simulink library "Rishi_Library"  (R2023a)
settings: Solver=VariableStepAuto  StartTime=0.0  StopTime=10.0  RelTol=1e-3

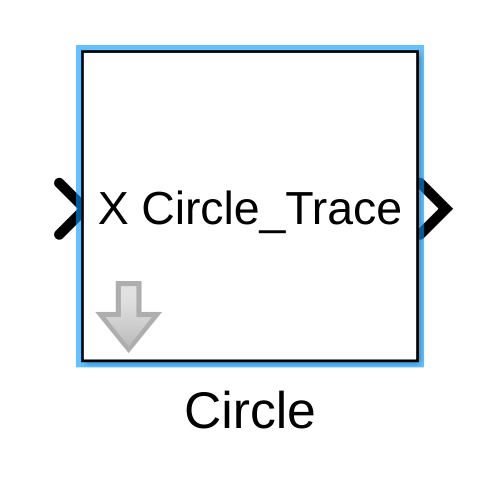
[thumbnail: Simulink's stored preview of the top-level diagram]
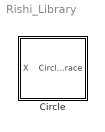
== system Rishi_Library ==
  Circle : Subsystem  mask{X_Offset=0, Y_Offset=0, Radius=0}
      mask prompts: X_Offset "X Offset"; Y_Offset "Y Offset"

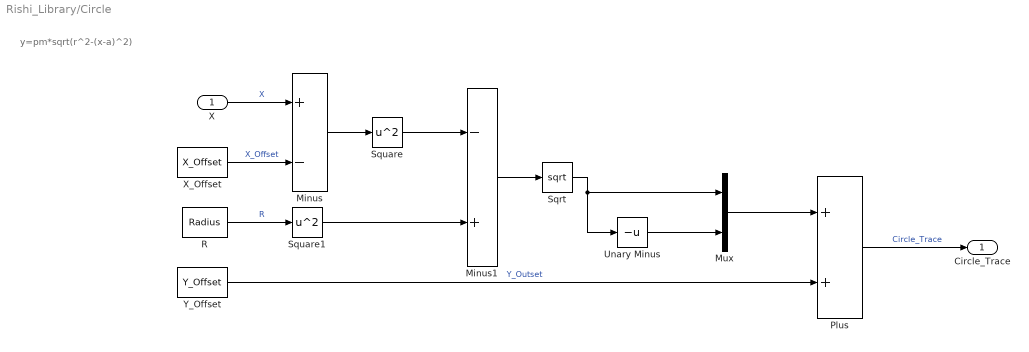
== system Rishi_Library/Circle ==
  note: y=pm*sqrt(r^2-(x-a)^2)
  X : Inport
  Minus : Sum  Inputs=+-
  Minus1 : Sum  Inputs=-+
  Mux : Mux  Inputs=2
  Plus : Sum
  R : Constant  Value=Radius
  Sqrt : Sqrt
  Square : Math  Operator=square
  Square1 : Math  Operator=square
  Unary Minus : UnaryMinus
  X_Offset : Constant  Value=X_Offset
  Y_Offset : Constant  Value=Y_Offset
  Circle_Trace : Outport
  wires:
  Square/1 -> Minus1/1
  Minus1/1 -> Sqrt/1
  Minus/1 -> Square/1
  Y_Offset/1 -> Plus/2  "Y_Outset"
  X/1 -> Minus/1  "X"
  Sqrt/1 -> Unary Minus/1, Mux/1
  Square1/1 -> Minus1/2
  Mux/1 -> Plus/1
  Unary Minus/1 -> Mux/2
  R/1 -> Square1/1  "R"
  X_Offset/1 -> Minus/2  "X_Offset"
  Plus/1 -> Circle_Trace/1  "Circle_Trace"
